simulink model "Subsys1NoActions"  (Simulink 9.0)
settings: Solver=FixedStepDiscrete  StartTime=0.0  StopTime=10.0  RelTol=1e-3  EnableMultiTasking=on
settings Model: SuppressorTable=22 serialization::archive 11 0 6 0 0 0 0 0  Creator=sofronis  LastModifiedBy=ktrinh  ExtModeAutoUpdateStatusClock=off
settings DataIOCC: LimitDataPoints=on  SignalLoggingSaveFormat=ModelDataLogs  SignalLoggingName=sigsOut
settings DebuggingCC: AlgebraicLoopMsg=error  SaveWithParameterizedLinksMsg=none  SignalResolutionControl=TryResolveAllWithWarning  MultiTaskDSMMsg=warning  MultiTaskCondExecSysMsg=none
settings HardwareCC: TargetUnknown=on
settings SFSimCC: SimParseCustomCode=off
settings GRTTargetCC: CombineOutputUpdateFcns=off  GRTInterface=on

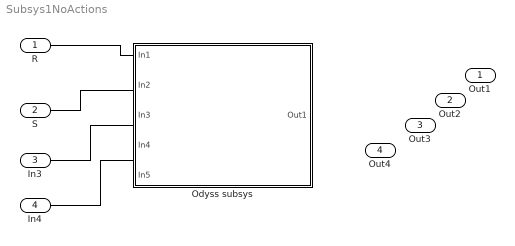
== system Subsys1NoActions ==
  R : Inport  SampleTime=1
  S : Inport  Port=2  SampleTime=1
  In3 : Inport  Port=3  SampleTime=1
  In4 : Inport  Port=4  SampleTime=1
  Odyss subsys : Subsystem
  Out1 : Outport
  Out2 : Outport  Port=2
  Out3 : Outport  Port=3
  Out4 : Outport  Port=4
  wires:
  R/1 -> ?
  S/1 -> ?
  In3/1 -> ?
  In4/1 -> ?
  ? -> Out1/1
  ? -> Out2/1
  ? -> Out3/1
  ? -> Out4/1

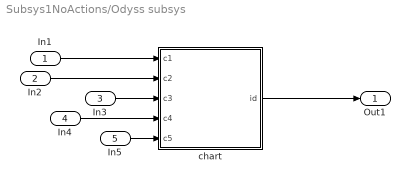
== system Subsys1NoActions/Odyss subsys ==
  In1 : Inport  OutDataTypeStr=boolean
  In2 : Inport  Port=2  OutDataTypeStr=boolean
  In3 : Inport  Port=3  OutDataTypeStr=boolean
  In4 : Inport  Port=4  OutDataTypeStr=boolean
  In5 : Inport  Port=5  OutDataTypeStr=boolean
  chart : Stateflow chart  TreatAsAtomicUnit=on
  Out1 : Outport
  wires:
  chart/1(id) -> Out1/1
  In1/1 -> chart/1(c1)
  In5/1 -> chart/5(c5)
  In4/1 -> chart/4(c4)
  In3/1 -> chart/3(c3)
  In2/1 -> chart/2(c2)

== stateflow chart Odyss subsys/chart ==
  state A [parallel]
    settings: executionOrder=1
    state Aa/
      en:id=1;
    state Ab/
      en:id=2;
    (default) -> Aa
    Aa -> Ab : [c2]
    Ab -> Aa : [c1]
  state B [parallel]
    settings: executionOrder=2
    state Ba/
      en:id=3;
    state Bb/
      en:id=4;
    (default) -> Ba
    Ba -> Bb : [c5]
    Bb -> Ba : [c4]
  state C [parallel]
    settings: executionOrder=3
    state Ca/
      en:id=5;
    state Cb/
      en:id=6;
    (default) -> Ca
    Ca -> Cb : [c1]
    Cb -> Ca : [c2]
  state D [parallel]
    settings: executionOrder=4
    state Da/
      en:id=7;
    state Db/
      en:id=8;
    (default) -> Da
    Da -> Db : [c3]
    Db -> Da : [c3]
  data: c1 input double; c2 input double; c3 input double; c4 input double; c5 input double; id output double
